simulink model "RST_Sami_Fahim_R2022a"  (R2022a)
settings: Solver=ode1  StartTime=0.0  StopTime=0.05  FixedStep=1e-7  RelTol=1e-3
undefined symbols (not defined in the file): Te
libraries: cstblocks x5, dspsrcs4 x3
settings Model: Creator=vlechappe  LastModifiedBy=sfahim
settings SolverCC: AlgebraicLoopSolver=TrustRegion
settings DebuggingCC: UnconnectedInputMsg=warning  UnconnectedOutputMsg=warning  UnconnectedLineMsg=warning
settings SFSimCC: CustomCodeUndefinedFunction=UseInterfaceOnly

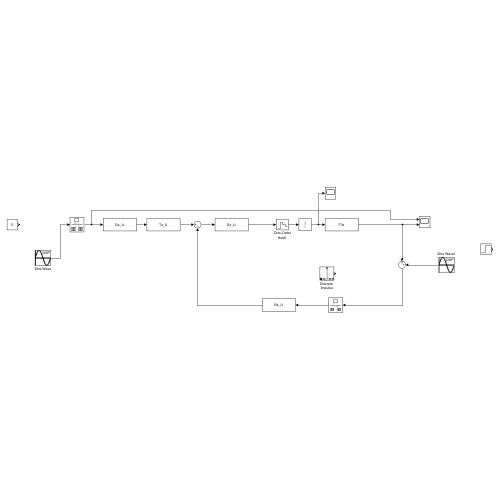
[thumbnail: Simulink's stored preview of the top-level diagram]
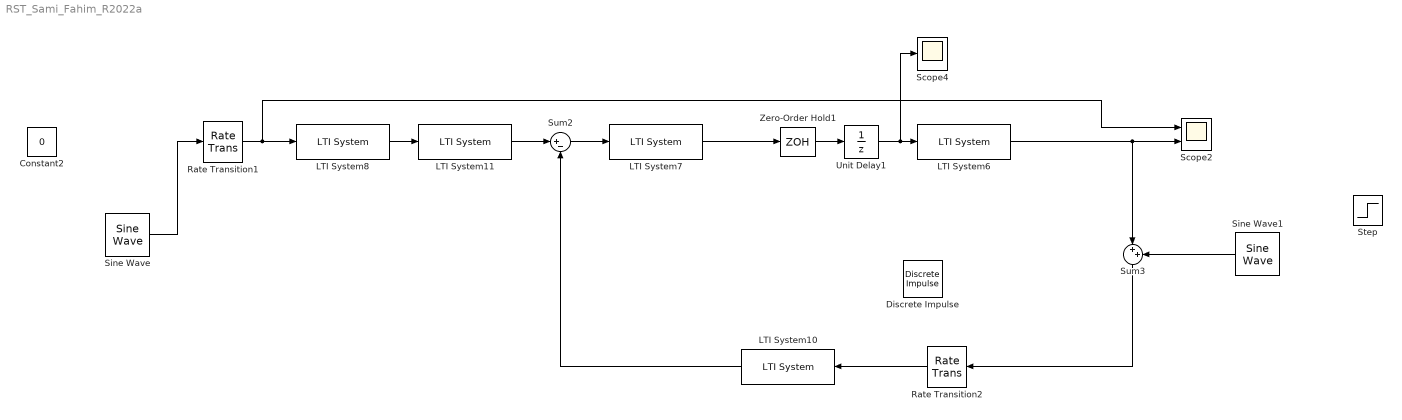
== system RST_Sami_Fahim_R2022a ==
  Constant2 : Constant  Value=0  SampleTime=Te
  Discrete Impulse : dspsrcs4/Discrete  Impulse  Delay=0  SampleTime=1  FrameSample=1  OutputFrames=off  dataType=double  isSigned=on  wordLen=16  udDataType=sfix(16)  fracBitsMode=Best precision  numFracBits=15  OutDataTypeStr=double  LastOutDataTypeStr=double
  LTI System10 : cstblocks/LTI System  sys=Rz_U  IC=[]
  LTI System11 : cstblocks/LTI System  sys=Tz_U  IC=[]
  LTI System6 : cstblocks/LTI System  sys=F3z  IC=[]
  LTI System7 : cstblocks/LTI System  sys=Sz_U  IC=[]
  LTI System8 : cstblocks/LTI System  sys=Gz_U  IC=[]
  Rate Transition1 : RateTransition  OutPortSampleTime=Te
  Rate Transition2 : RateTransition  OutPortSampleTime=Te
  Scope2 : Scope  NumInputPorts=2
  Scope4 : Scope
  Sine Wave : dspsrcs4/Sine Wave  Amplitude=230  Frequency=50  Phase=0  SampleMode=Continuous  OutComplex=Real  CompMethod=Trigonometric fcn  TableSize=Speed  SampleTime=1/1000  SamplesPerFrame=1  ResetState=Restart at time zero  OutputFrames=off  dataType=double  wordLen=16  udDataType=sfix(16)  fracBitsMode=Best precision  numFracBits=15  OutDataTypeStr=double  LastOutDataTypeStr=double
  Sine Wave1 : dspsrcs4/Sine Wave  Amplitude=10  Frequency=150  Phase=0  SampleMode=Continuous  OutComplex=Real  CompMethod=Trigonometric fcn  TableSize=Speed  SampleTime=1/1000  SamplesPerFrame=1  ResetState=Restart at time zero  OutputFrames=off  dataType=double  wordLen=16  udDataType=sfix(16)  fracBitsMode=Best precision  numFracBits=15  OutDataTypeStr=double  LastOutDataTypeStr=double
  Step : Step  Time=0.03  After=10  SampleTime=0
  Sum2 : Sum  Inputs=|+-
  Sum3 : Sum  Inputs=|++
  Unit Delay1 : UnitDelay  SampleTime=-1  HasFrameUpgradeWarning=on
  Zero-Order Hold1 : ZeroOrderHold  SampleTime=Te
  wires:
  Rate Transition1/1 -> Scope2/1, LTI System8/1
  Unit Delay1/1 -> Scope4/1, LTI System6/1
  Zero-Order Hold1/1 -> Unit Delay1/1
  Sum2/1 -> LTI System7/1
  LTI System7/1 -> Zero-Order Hold1/1
  LTI System10/1 -> Sum2/2
  LTI System8/1 -> LTI System11/1
  LTI System11/1 -> Sum2/1
  Rate Transition2/1 -> LTI System10/1
  LTI System6/1 -> Sum3/1, Scope2/2
  Sine Wave/1 -> Rate Transition1/1
  Sum3/1 -> Rate Transition2/1
  Sine Wave1/1 -> Sum3/2
